simulink model "Flight_simulator_nl"  (R2025b)
settings: Solver=ode4  StartTime=0.0  StopTime=300  FixedStep=0.02  RelTol=1e-3
InitFcn:
  | navion_params;
  | actuator_params;
  | figs0 = findall(0, 'type', 'figure');
  | vis0  = get(0, 'DefaultFigureVisible');
  | set(0, 'DefaultFigureVisible', 'off');
  | evalc('longitudinal_pitch_control; lateral_directional_control;');
  | set(0, 'DefaultFigureVisible', vis0);
  | close(setdiff(findall(0, 'type', 'figure'), figs0));
  | if ~exist('fb_on',   'var'), fb_on   = 1; end
  | if ~exist('gust_on', 'var'), gust_on = 1; end
  | if ~exist('trk_on','var'), trk_on = 1; end
  | nl_setup;
undefined symbols (not defined in the file): act_on, alt_on, F, fb_on, gust_on, Kh, Ki, Kp, Kphi, Kpsi, Kq, Kv, Kvi, Kxi, Ky, Kzeta, Light, MIL, nl_x0, pos_ail, pos_ele, pos_rud, psi_int_lim, sens_on, tau_sens, tau_thr, trk_on, V0
libraries: aerolibactuator x3, slpidlib x2, aerolibwind2 x1
settings Model: Creator=USER  LastModifiedBy=USER

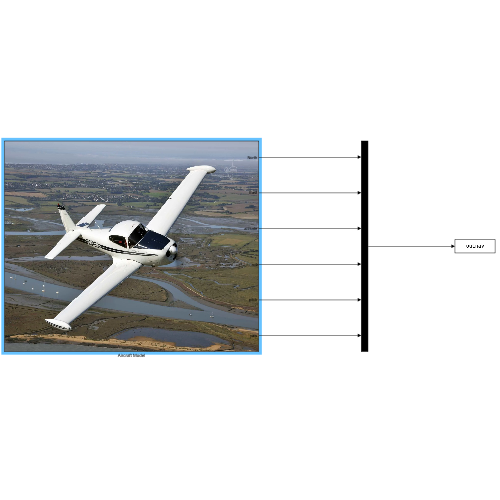
[thumbnail: Simulink's stored preview of the top-level diagram]
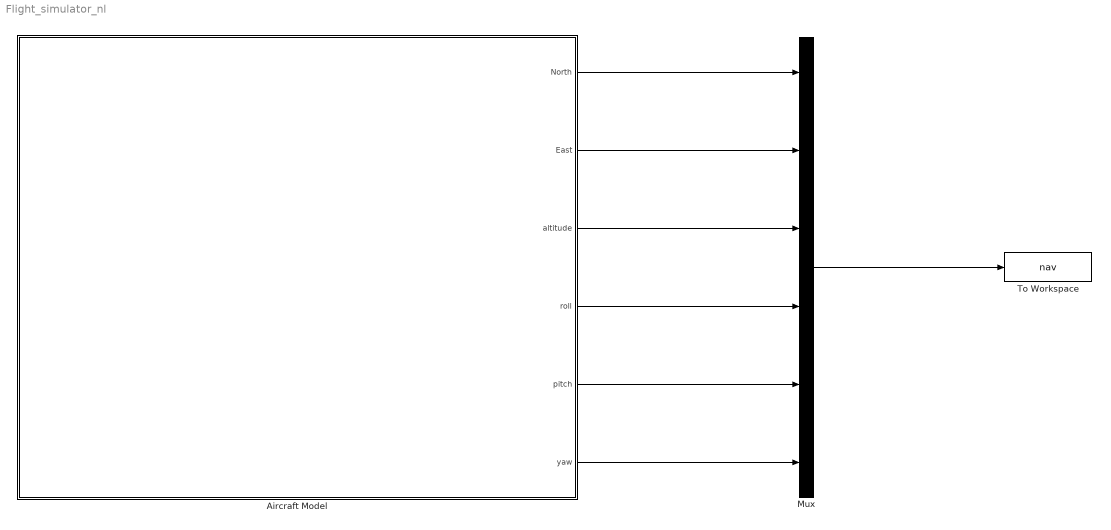
== system Flight_simulator_nl ==
  Aircraft Model : Subsystem
      mask Display: image('img.webp');
  Mux : Mux  Inputs=6
  To Workspace : ToWorkspace  VariableName=nav  SampleTime=-1
  wires:
  Aircraft Model/4(roll) -> Mux/4
  Aircraft Model/5(pitch) -> Mux/5
  Aircraft Model/6(yaw) -> Mux/6
  Aircraft Model/2(East) -> Mux/2
  Aircraft Model/1(North) -> Mux/1
  Aircraft Model/3(altitude) -> Mux/3
  Mux/1 -> To Workspace/1

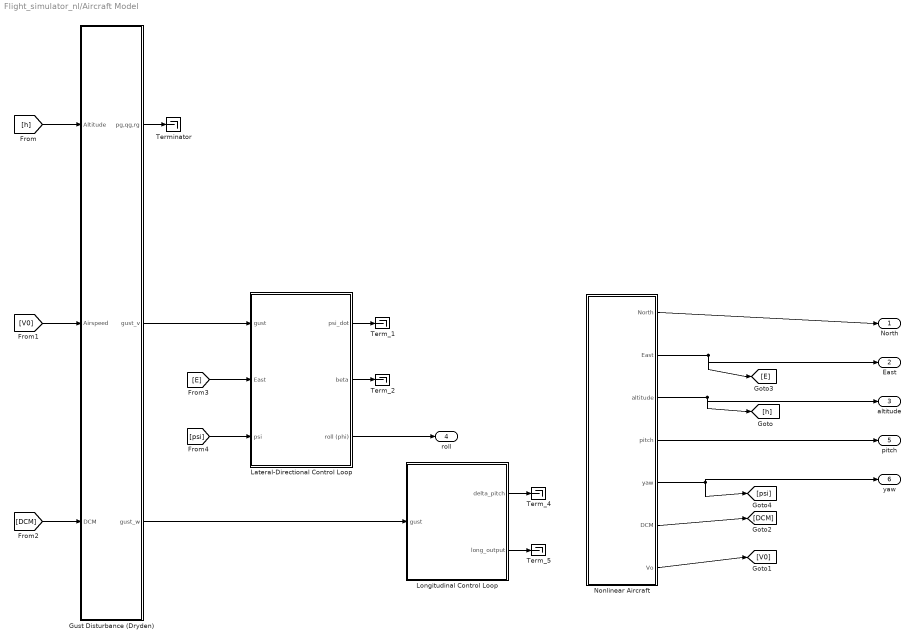
== system Flight_simulator_nl/Aircraft Model ==
  Gust Disturbance (Dryden) : Subsystem
  Lateral-Directional Control Loop : Subsystem
  Longitudinal Control Loop : Subsystem
  Nonlinear Aircraft : Subsystem
  Term_{1..2,4..5} (4 alike) : Terminator
  Terminator : Terminator
  North : Outport
  East : Outport  Port=2
  altitude : Outport  Port=3
  roll : Outport  Port=4
  pitch : Outport  Port=5
  yaw : Outport  Port=6
  wires:
  Gust Disturbance (Dryden)/3(gust_w) -> Longitudinal Control Loop/1(gust)
  [DCM] -> Gust Disturbance (Dryden)/3(DCM)
  [h] -> Gust Disturbance (Dryden)/1(Altitude)
  [V0] -> Gust Disturbance (Dryden)/2(Airspeed)
  Lateral-Directional Control Loop/3(roll (phi)) -> roll/1
  Gust Disturbance (Dryden)/1(pg,qg,rg) -> Terminator/1
  Gust Disturbance (Dryden)/2(gust_v) -> Lateral-Directional Control Loop/1(gust)
  [E] -> Lateral-Directional Control Loop/2(East)
  [psi] -> Lateral-Directional Control Loop/3(psi)
  Lateral-Directional Control Loop/1(psi_dot) -> Term_1/1
  Lateral-Directional Control Loop/2(beta) -> Term_2/1
  Longitudinal Control Loop/1("delta_pitch ") -> Term_4/1
  Longitudinal Control Loop/2(long_output) -> Term_5/1
  Nonlinear Aircraft/1(North) -> North/1
  Nonlinear Aircraft/2(East) -> [E], East/1
  Nonlinear Aircraft/3(altitude) -> [h], altitude/1
  Nonlinear Aircraft/4(pitch) -> pitch/1
  Nonlinear Aircraft/5(yaw) -> [psi], yaw/1
  Nonlinear Aircraft/6(DCM) -> [DCM]
  Nonlinear Aircraft/7(Vo) -> [V0]

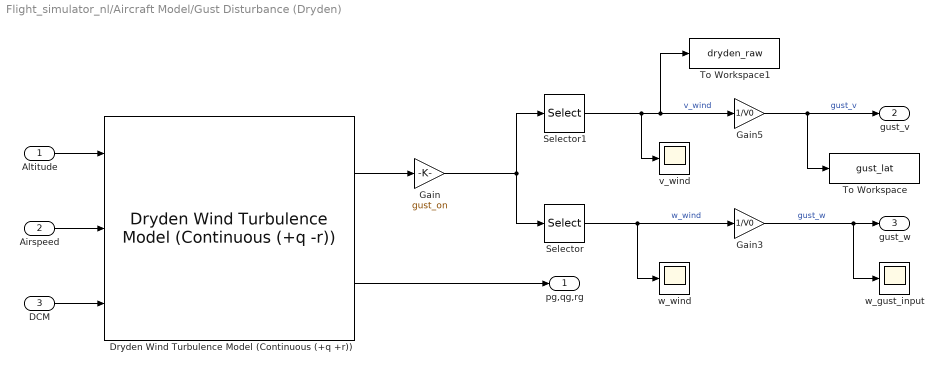
== system Flight_simulator_nl/Aircraft Model/Gust Disturbance (Dryden) ==
  Altitude : Inport
  Airspeed : Inport  Port=2
  DCM : Inport  Port=3
  Dryden Wind Turbulence Model (Continuous (+q +r)) : aerolibwind2/Dryden Wind Turbulence Model  (Continuous (+q -r))  units=Metric (MKS)  spec=MIL-F-8785C  model=Continuous Dryden (+q +r)  W20=15  Wdeg=0  TurbProb=10^-2 - Light  L_high=533.4  Wingspan=10  ts=0.1  Seed=[1010 1011 1012 1013]  T_on=on
      settings: LibrarySourceBlock=|
      | aerolibwind2/Dryden Wind Turbulence Model
      | (Continuous (+q +r))
  Gain : Gain  Gain=gust_on
  Gain3 : Gain  Gain=1/V0
  Gain5 : Gain  Gain=1/V0
  Selector : Selector  InputPortWidth=3  IndexOptions=Index vector (dialog)  Indices=3  OutputSizes=1
  Selector1 : Selector  InputPortWidth=3  IndexOptions=Index vector (dialog)  Indices=2  OutputSizes=1
  To Workspace : ToWorkspace  VariableName=gust_lat  SampleTime=-1
  To Workspace1 : ToWorkspace  VariableName=dryden_raw  SampleTime=-1
  v_wind : Scope
      settings: ActiveDisplayYMinimum=-2.1718299710396272  ActiveDisplayYMaximum=2.2933542366070889  DataLoggingVariableName=ScopeData3
  w_gust_input : Scope
      settings: ActiveDisplayYMinimum=-10.465820831986111  ActiveDisplayYMaximum=10.534179168013885
  w_wind : Scope
      settings: ActiveDisplayYMinimum=-10.465820831986111  ActiveDisplayYMaximum=10.534179168013885  DataLoggingVariableName=ScopeData2
  pg,qg,rg : Outport
  gust_v : Outport  Port=2
  gust_w : Outport  Port=3
  wires:
  Selector1/1 -> v_wind/1, To Workspace1/1, Gain5/1  "v_wind"
  Altitude/1 -> Dryden Wind Turbulence Model (Continuous (+q +r))/1
  Airspeed/1 -> Dryden Wind Turbulence Model (Continuous (+q +r))/2
  Dryden Wind Turbulence Model (Continuous (+q +r))/2 -> pg,qg,rg/1
  DCM/1 -> Dryden Wind Turbulence Model (Continuous (+q +r))/3
  Dryden Wind Turbulence Model (Continuous (+q +r))/1 -> Gain/1
  Selector/1 -> Gain3/1, w_wind/1  "w_wind"
  Gain5/1 -> To Workspace/1, gust_v/1  "gust_v"
  Gain3/1 -> gust_w/1, w_gust_input/1  "gust_w"
  Gain/1 -> Selector/1, Selector1/1

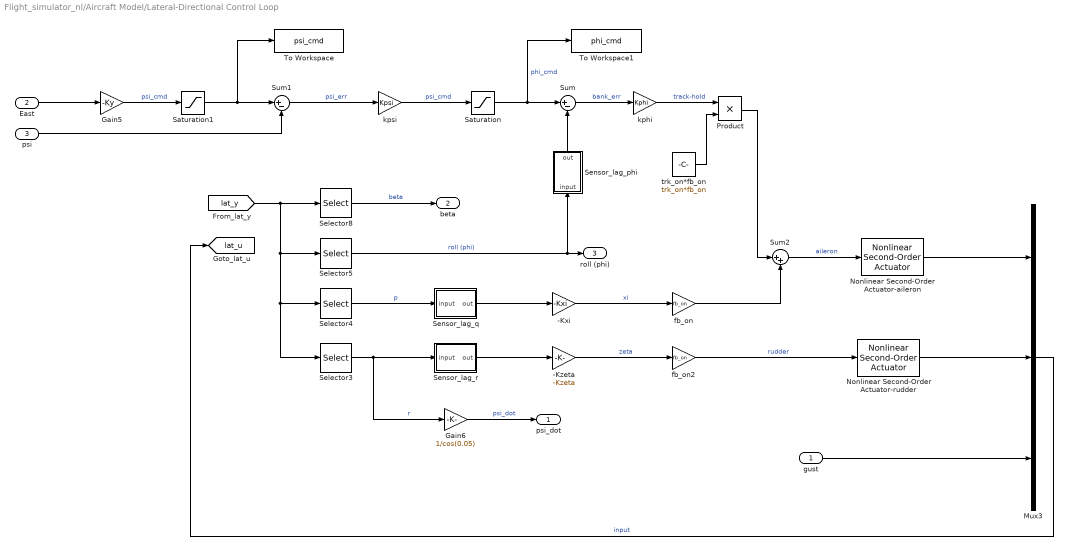
== system Flight_simulator_nl/Aircraft Model/Lateral-Directional Control Loop ==
  gust : Inport
  East : Inport  Port=2
  psi : Inport  Port=3
  -Kxi : Gain  Gain=-Kxi
  -Kzeta : Gain  Gain=-Kzeta
  Gain5 : Gain  Gain=-Ky
  Gain6 : Gain  Gain=1/cos(0.05)
  Mux3 : Mux  Inputs=3
  Nonlinear Second-Order Actuator-aileron : aerolibactuator/Nonlinear Second-Order Actuator  wn_fin=wn_ail  z_fin=zeta_ail  fin_max=pos_ail  fin_min=-pos_ail  fin_maxrate=rate_ail  fin_act_0=0  fin_act_vel=0
  Nonlinear Second-Order Actuator-rudder : aerolibactuator/Nonlinear Second-Order Actuator  wn_fin=wn_rud  z_fin=zeta_rud  fin_max=pos_rud  fin_min=-pos_rud  fin_maxrate=rate_rud  fin_act_0=0  fin_act_vel=0
  Product : Product
  Saturation : Saturate  UpperLimit=0.35  LowerLimit=-0.35
  Saturation1 : Saturate  UpperLimit=psi_int_lim  LowerLimit=-psi_int_lim
  Selector3 : Selector  InputPortWidth=4  IndexOptions=Index vector (dialog)  Indices=1  OutputSizes=1
  Selector4 : Selector  InputPortWidth=4  IndexOptions=Index vector (dialog)  Indices=3  OutputSizes=1
  Selector5 : Selector  InputPortWidth=4  IndexOptions=Index vector (dialog)  Indices=4  OutputSizes=1
  Selector8 : Selector  InputPortWidth=4  IndexOptions=Index vector (dialog)  Indices=2  OutputSizes=1
  Sensor_lag_phi : Subsystem
  Sensor_lag_q : Subsystem
  Sensor_lag_r : Subsystem
  Sum : Sum  Inputs=|+-
  Sum1 : Sum  Inputs=|+-
  Sum2 : Sum  Inputs=|++
  To Workspace : ToWorkspace  VariableName=psi_cmd  SampleTime=-1
  To Workspace1 : ToWorkspace  VariableName=phi_cmd  SampleTime=-1
  fb_on : Gain  Gain=fb_on
  fb_on2 : Gain  Gain=fb_on
  kphi : Gain  Gain=Kphi
  kpsi : Gain  Gain=Kpsi
  trk_on*fb_on : Constant  Value=trk_on*fb_on
  psi_dot : Outport
  beta : Outport  Port=2
  roll (phi) : Outport  Port=3
  tag scope: lat_u=global
  wires:
  Selector4/1 -> Sensor_lag_q/1(input)  "p"
  Gain6/1 -> psi_dot/1  "psi_dot"
  Selector5/1 -> roll (phi)/1, Sensor_lag_phi/1(input)  "roll (phi)"
  Selector8/1 -> beta/1  "beta"
  gust/1 -> Mux3/3
  Selector3/1 -> Gain6/1, Sensor_lag_r/1(input)  "r"
  -Kxi/1 -> fb_on/1  "xi"
  -Kzeta/1 -> fb_on2/1  "zeta"
  fb_on/1 -> Sum2/2
  fb_on2/1 -> Nonlinear Second-Order Actuator-rudder/1  "rudder"
  Gain5/1 -> Saturation1/1  "psi_cmd"
  Sum1/1 -> kpsi/1  "psi_err"
  kpsi/1 -> Saturation/1  "psi_cmd"
  East/1 -> Gain5/1
  Saturation/1 -> To Workspace1/1, Sum/1  "phi_cmd"
  Sum/1 -> kphi/1  "bank_err"
  kphi/1 -> Product/1  "track-hold"
  Sum2/1 -> Nonlinear Second-Order Actuator-aileron/1  "aileron"
  Product/1 -> Sum2/1
  trk_on*fb_on/1 -> Product/2
  psi/1 -> Sum1/2
  Nonlinear Second-Order Actuator-rudder/1 -> Mux3/2
  Sensor_lag_q/1(out) -> -Kxi/1
  Sensor_lag_r/1(out) -> -Kzeta/1
  Sensor_lag_phi/1(out) -> Sum/2
  Nonlinear Second-Order Actuator-aileron/1 -> Mux3/1
  [lat_y] -> Selector8/1, Selector3/1, Selector4/1, Selector5/1
  Mux3/1 -> [lat_u]  "input"
  Saturation1/1 -> To Workspace/1, Sum1/1

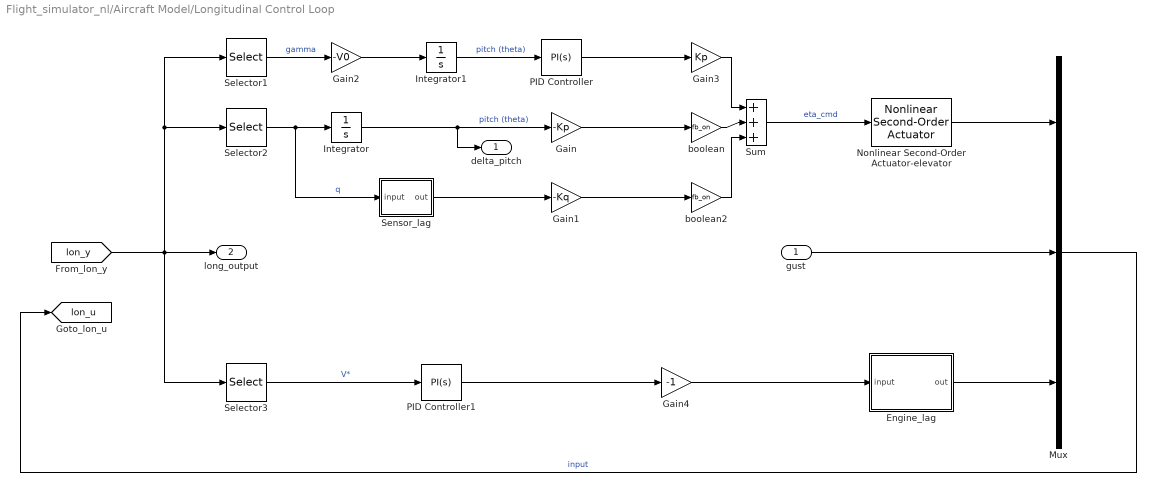
== system Flight_simulator_nl/Aircraft Model/Longitudinal Control Loop ==
  gust : Inport
  Engine_lag : Subsystem  mask{tau=tau_thr, rate_lim=inf, pos_lim=inf}
      mask prompts: tau "Time constant [s]"; rate_lim "Rate limit [rad/s]"; pos_lim "Position limit [rad]"
  Gain : Gain  Gain=-Kp
  Gain1 : Gain  Gain=-Kq
  Gain2 : Gain  Gain=-V0
  Gain3 : Gain  Gain=Kp
  Gain4 : Gain  Gain=-1
  Integrator : Integrator
  Integrator1 : Integrator
  Mux : Mux  Inputs=3
  Nonlinear Second-Order Actuator-elevator : aerolibactuator/Nonlinear Second-Order Actuator  wn_fin=wn_ele  z_fin=zeta_ele  fin_max=pos_ele  fin_min=-pos_ele  fin_maxrate=rate_ele  fin_act_0=0  fin_act_vel=0
  PID Controller : slpidlib/PID Controller  Controller=PI  Form=Parallel  TimeDomain=Continuous-time  UseExternalTs=off  SampleTime=-1  IntegratorMethod=Forward Euler  FilterMethod=Forward Euler  ControllerParametersSource=internal  P=Kh*alt_on  I=Ki*alt_on  UseKiTs=off  D=0  UseExternalDerivativeSource=off  N=100  UseFilter=on  TunerSelectOption=Transfer Function Based (PID Tuner App)  InitialConditionSource=internal  InitialConditionForIntegrator=0  InitialConditionForFilter=0  DifferentiatorICPrevScaledInput=0  ExternalReset=none  TrackingMode=off  Kt=1  LimitOutput=off  SatLimitsSource=internal  UpperSaturationLimit=inf  LowerSaturationLimit=-inf  LinearizeAsGain=on  AntiWindupMode=none  Kb=1  LimitIntegrator=off  UpperIntegratorSaturationLimit=inf  LowerIntegratorSaturationLimit=-inf  POutMin=[]  POutMax=[]  IOutMin=[]  IOutMax=[]  DOutMin=[]  DOutMax=[]  NOutMin=[]  NOutMax=[]  SumOutMin=[]  SumOutMax=[]  SaturationOutMin=[]  SaturationOutMax=[]  PParamMin=[]  PParamMax=[]  IParamMin=[]  IParamMax=[]  DParamMin=[]  DParamMax=[]  NParamMin=[]  NParamMax=[]  KbParamMin=[]  KbParamMax=[]  KtParamMin=[]  KtParamMax=[]  KbOutMin=[]  KbOutMax=[]  KtOutMin=[]  KtOutMax=[]  IntegratorOutMin=[]  IntegratorOutMax=[]  FilterOutMin=[]  FilterOutMax=[]  SumI1OutMin=[]  SumI1OutMax=[]  SumI2OutMin=[]  SumI2OutMax=[]  SumI3OutMin=[]  SumI3OutMax=[]  SumI4OutMin=[]  SumI4OutMax=[]  SumDOutMin=[]  SumDOutMax=[]  DifferentiatorOutMin=[]  DifferentiatorOutMax=[]  FilterDiffOutCoefMin=[]  FilterDiffOutCoefMax=[]  ReciprocalOutMin=[]  ReciprocalOutMax=[]  SumDenOutMin=[]  SumDenOutMax=[]  SumNumOutMin=[]  SumNumOutMax=[]  DivideOutMin=[]  DivideOutMax=[]  UdiffTsProdOutMin=[]  UdiffTsProdOutMax=[]  NTsProdOutMin=[]  NTsProdOutMax=[]  UintegralTsProdOutMin=[]  UintegralTsProdOutMax=[]  UngainTsProdOutMin=[]  UngainTsProdOutMax=[]  ClampingZeroOutDataTypeStr=Inherit: Inherit via back propagation  ClampingZeroOutMin=[]  ClampingZeroOutMax=[]  FilterDenConstantOutDataTypeStr=Inherit: Inherit via back propagation  FilterDenConstantOutMin=[]  FilterDenConstantOutMax=[]  PCopyOutDataTypeStr=Inherit: Inherit via back propagation  PCopyOutMin=[]  PCopyOutMax=[]  NCopyOutDataTypeStr=Inherit: Inherit via back propagation  NCopyOutMin=[]  NCopyOutMax=[]  IntegratorContinuousStateAttributes=''  IntegratorStateMustResolveToSignalObject=off  IntegratorRTWStateStorageClass=Auto  FilterContinuousStateAttributes=''  FilterStateMustResolveToSignalObject=off  FilterRTWStateStorageClass=Auto  ParallelPVariant=InternalParameters  IdealPVariant=Disabled  IVariant=InternalParameters  DVariant=Disabled  IntegratorVariant=Continuous  SatVariant=Disabled  AWVariant=Passthrough  PCopyVariant=Disabled  TRVariant=Disabled  FdbkBlocksVariant=Forward  IdealPFdbkVariant=Disabled  SatFdbkVariant=Disabled  DerivativeFilterVariant=Disabled  NVariant=Disabled  NCopyVariant=Disabled_SignalSpec  FilterICVariant=Disabled  IntegratorICVariant=InternalICs  ExternalResetVariant=Disabled  TRSumVariant=Passthrough  SumFdbkVariant=Disabled  SumVariant=Sum_PI  TsampFilterVariant=InternalTs  TsampNgainVariant=Passthrough  TsampIntegralVariant=Disabled_SignalSpec  ExternalSaturationOutDataTypeStr=Inherit: Same as second input  DerivativeSourceVariant=Disabled  PreIntVariant=InternalPreInt
  PID Controller1 : slpidlib/PID Controller  Controller=PI  Form=Parallel  TimeDomain=Continuous-time  UseExternalTs=off  SampleTime=-1  IntegratorMethod=Forward Euler  FilterMethod=Forward Euler  ControllerParametersSource=internal  P=Kv*alt_on  I=Kvi*alt_on  UseKiTs=off  D=0  UseExternalDerivativeSource=off  N=100  UseFilter=on  TunerSelectOption=Transfer Function Based (PID Tuner App)  InitialConditionSource=internal  InitialConditionForIntegrator=0  InitialConditionForFilter=0  DifferentiatorICPrevScaledInput=0  ExternalReset=none  TrackingMode=off  Kt=1  LimitOutput=off  SatLimitsSource=internal  UpperSaturationLimit=inf  LowerSaturationLimit=-inf  LinearizeAsGain=on  AntiWindupMode=none  Kb=1  LimitIntegrator=off  UpperIntegratorSaturationLimit=inf  LowerIntegratorSaturationLimit=-inf  POutMin=[]  POutMax=[]  IOutMin=[]  IOutMax=[]  DOutMin=[]  DOutMax=[]  NOutMin=[]  NOutMax=[]  SumOutMin=[]  SumOutMax=[]  SaturationOutMin=[]  SaturationOutMax=[]  PParamMin=[]  PParamMax=[]  IParamMin=[]  IParamMax=[]  DParamMin=[]  DParamMax=[]  NParamMin=[]  NParamMax=[]  KbParamMin=[]  KbParamMax=[]  KtParamMin=[]  KtParamMax=[]  KbOutMin=[]  KbOutMax=[]  KtOutMin=[]  KtOutMax=[]  IntegratorOutMin=[]  IntegratorOutMax=[]  FilterOutMin=[]  FilterOutMax=[]  SumI1OutMin=[]  SumI1OutMax=[]  SumI2OutMin=[]  SumI2OutMax=[]  SumI3OutMin=[]  SumI3OutMax=[]  SumI4OutMin=[]  SumI4OutMax=[]  SumDOutMin=[]  SumDOutMax=[]  DifferentiatorOutMin=[]  DifferentiatorOutMax=[]  FilterDiffOutCoefMin=[]  FilterDiffOutCoefMax=[]  ReciprocalOutMin=[]  ReciprocalOutMax=[]  SumDenOutMin=[]  SumDenOutMax=[]  SumNumOutMin=[]  SumNumOutMax=[]  DivideOutMin=[]  DivideOutMax=[]  UdiffTsProdOutMin=[]  UdiffTsProdOutMax=[]  NTsProdOutMin=[]  NTsProdOutMax=[]  UintegralTsProdOutMin=[]  UintegralTsProdOutMax=[]  UngainTsProdOutMin=[]  UngainTsProdOutMax=[]  ClampingZeroOutDataTypeStr=Inherit: Inherit via back propagation  ClampingZeroOutMin=[]  ClampingZeroOutMax=[]  FilterDenConstantOutDataTypeStr=Inherit: Inherit via back propagation  FilterDenConstantOutMin=[]  FilterDenConstantOutMax=[]  PCopyOutDataTypeStr=Inherit: Inherit via back propagation  PCopyOutMin=[]  PCopyOutMax=[]  NCopyOutDataTypeStr=Inherit: Inherit via back propagation  NCopyOutMin=[]  NCopyOutMax=[]  IntegratorContinuousStateAttributes=''  IntegratorStateMustResolveToSignalObject=off  IntegratorRTWStateStorageClass=Auto  FilterContinuousStateAttributes=''  FilterStateMustResolveToSignalObject=off  FilterRTWStateStorageClass=Auto  ParallelPVariant=InternalParameters  IdealPVariant=Disabled  IVariant=InternalParameters  DVariant=Disabled  IntegratorVariant=Continuous  SatVariant=Disabled  AWVariant=Passthrough  PCopyVariant=Disabled  TRVariant=Disabled  FdbkBlocksVariant=Forward  IdealPFdbkVariant=Disabled  SatFdbkVariant=Disabled  DerivativeFilterVariant=Disabled  NVariant=Disabled  NCopyVariant=Disabled_SignalSpec  FilterICVariant=Disabled  IntegratorICVariant=InternalICs  ExternalResetVariant=Disabled  TRSumVariant=Passthrough  SumFdbkVariant=Disabled  SumVariant=Sum_PI  TsampFilterVariant=InternalTs  TsampNgainVariant=Passthrough  TsampIntegralVariant=Disabled_SignalSpec  ExternalSaturationOutDataTypeStr=Inherit: Same as second input  DerivativeSourceVariant=Disabled  PreIntVariant=InternalPreInt
  Selector1 : Selector  InputPortWidth=5  IndexOptions=Index vector (dialog)  Indices=2  OutputSizes=1
  Selector2 : Selector  InputPortWidth=5  IndexOptions=Index vector (dialog)  Indices=4  OutputSizes=1
  Selector3 : Selector  InputPortWidth=5  IndexOptions=Index vector (dialog)  Indices=1  OutputSizes=1
  Sensor_lag : Subsystem
  Sum : Sum  Inputs=|+++
  boolean : Gain  Gain=fb_on
  boolean2 : Gain  Gain=fb_on
  "delta_pitch " : Outport
  long_output : Outport  Port=2
  tag scope: lon_u=global
  wires:
  Selector2/1 -> Sensor_lag/1(input), Integrator/1  "q"
  Integrator/1 -> Gain/1, "delta_pitch "/1  "pitch (theta)"
  Sum/1 -> Nonlinear Second-Order Actuator-elevator/1  "eta_cmd"
  gust/1 -> Mux/2
  Gain1/1 -> boolean2/1
  Gain/1 -> boolean/1
  boolean/1 -> Sum/2
  boolean2/1 -> Sum/3
  Selector1/1 -> Gain2/1  "gamma"
  Gain2/1 -> Integrator1/1
  Integrator1/1 -> PID Controller/1  "pitch (theta)"
  Gain3/1 -> Sum/1
  PID Controller/1 -> Gain3/1
  Selector3/1 -> PID Controller1/1  "V*"
  PID Controller1/1 -> Gain4/1
  Gain4/1 -> Engine_lag/1(input)
  Nonlinear Second-Order Actuator-elevator/1 -> Mux/1
  Engine_lag/1(out) -> Mux/3
  Sensor_lag/1(out) -> Gain1/1
  [lon_y] -> Selector3/1, long_output/1, Selector2/1, Selector1/1
  Mux/1 -> [lon_u]  "input"

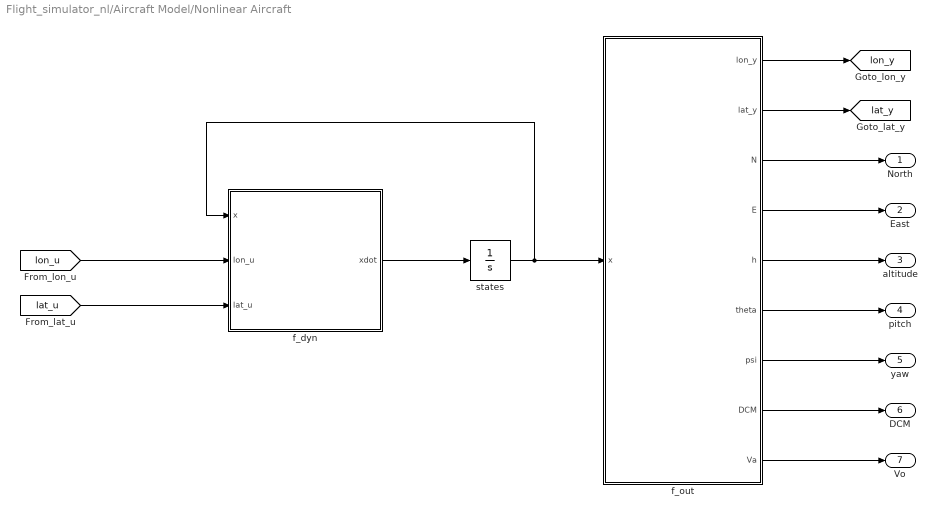
== system Flight_simulator_nl/Aircraft Model/Nonlinear Aircraft ==
  f_dyn : MATLAB Function  TreatAsAtomicUnit=on
  f_out : MATLAB Function  TreatAsAtomicUnit=on
  states : Integrator  InitialCondition=nl_x0
  North : Outport
  East : Outport  Port=2
  altitude : Outport  Port=3
  pitch : Outport  Port=4
  yaw : Outport  Port=5
  DCM : Outport  Port=6
  Vo : Outport  Port=7
  tag scope: lat_y=global, lon_y=global
  wires:
  states/1 -> f_out/1(x), f_dyn/1(x)
  [lon_u] -> f_dyn/2(lon_u)
  [lat_u] -> f_dyn/3(lat_u)
  f_dyn/1(xdot) -> states/1
  f_out/1(lon_y) -> [lon_y]
  f_out/2(lat_y) -> [lat_y]
  f_out/3(N) -> North/1
  f_out/4(E) -> East/1
  f_out/5(h) -> altitude/1
  f_out/6(theta) -> pitch/1
  f_out/7(psi) -> yaw/1
  f_out/8(DCM) -> DCM/1
  f_out/9(Va) -> Vo/1

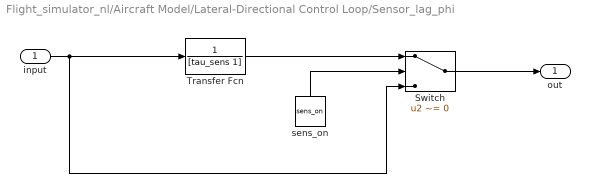
== system Flight_simulator_nl/Aircraft Model/Lateral-Directional Control Loop/Sensor_lag_phi ==
  input : Inport
  Switch : Switch  Criteria=u2 ~= 0  SaturateOnIntegerOverflow=off  InputSameDT=off
  Transfer Fcn : TransferFcn  Denominator=[tau_sens 1]
  sens_on : Constant  Value=sens_on
  out : Outport
  wires:
  Transfer Fcn/1 -> Switch/1
  input/1 -> Transfer Fcn/1, Switch/3
  Switch/1 -> out/1
  sens_on/1 -> Switch/2

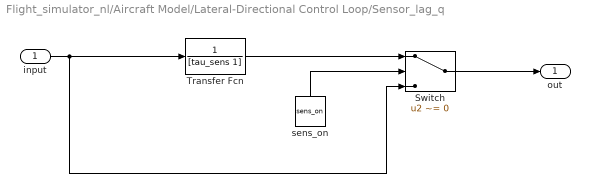
== system Flight_simulator_nl/Aircraft Model/Lateral-Directional Control Loop/Sensor_lag_q ==
  input : Inport
  Switch : Switch  Criteria=u2 ~= 0  SaturateOnIntegerOverflow=off  InputSameDT=off
  Transfer Fcn : TransferFcn  Denominator=[tau_sens 1]
  sens_on : Constant  Value=sens_on
  out : Outport
  wires:
  Transfer Fcn/1 -> Switch/1
  input/1 -> Transfer Fcn/1, Switch/3
  Switch/1 -> out/1
  sens_on/1 -> Switch/2

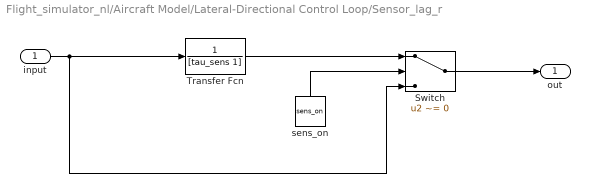
== system Flight_simulator_nl/Aircraft Model/Lateral-Directional Control Loop/Sensor_lag_r ==
  input : Inport
  Switch : Switch  Criteria=u2 ~= 0  SaturateOnIntegerOverflow=off  InputSameDT=off
  Transfer Fcn : TransferFcn  Denominator=[tau_sens 1]
  sens_on : Constant  Value=sens_on
  out : Outport
  wires:
  Transfer Fcn/1 -> Switch/1
  input/1 -> Transfer Fcn/1, Switch/3
  Switch/1 -> out/1
  sens_on/1 -> Switch/2

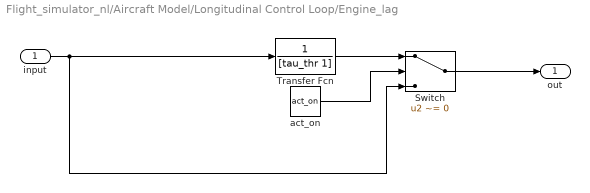
== system Flight_simulator_nl/Aircraft Model/Longitudinal Control Loop/Engine_lag ==
  input : Inport
  Switch : Switch  Criteria=u2 ~= 0  SaturateOnIntegerOverflow=off  InputSameDT=off
  Transfer Fcn : TransferFcn  Denominator=[tau_thr 1]
  act_on : Constant  Value=act_on
  out : Outport
  wires:
  Transfer Fcn/1 -> Switch/1
  input/1 -> Transfer Fcn/1, Switch/3
  Switch/1 -> out/1
  act_on/1 -> Switch/2

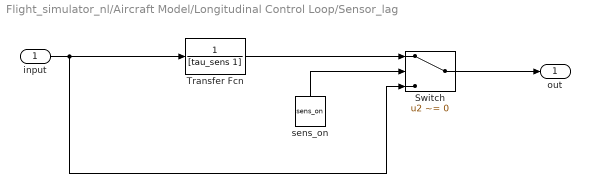
== system Flight_simulator_nl/Aircraft Model/Longitudinal Control Loop/Sensor_lag ==
  input : Inport
  Switch : Switch  Criteria=u2 ~= 0  SaturateOnIntegerOverflow=off  InputSameDT=off
  Transfer Fcn : TransferFcn  Denominator=[tau_sens 1]
  sens_on : Constant  Value=sens_on
  out : Outport
  wires:
  Transfer Fcn/1 -> Switch/1
  input/1 -> Transfer Fcn/1, Switch/3
  Switch/1 -> out/1
  sens_on/1 -> Switch/2

== matlab function Flight_simulator_nl/Aircraft Model/Nonlinear Aircraft/f_out ==
  data: x input size=12; lon_y output size=5; lat_y output size=4; N output size=1; E output size=1; h output size=1; theta output size=1; psi output size=1; DCM output size=[3 3]; Va output size=1
function [lon_y, lat_y, N, E, h, theta, psi, DCM, Va] = f_out(x)
P  = nl_const();
Vg = sqrt(x(1)^2 + x(2)^2 + x(3)^2);
st = sin(x(8)); ct = cos(x(8)); sp = sin(x(7)); cp = cos(x(7)); ss = sin(x(9)); cs = cos(x(9));
Rb2n = [ct*cs, sp*st*cs - cp*ss, cp*st*cs + sp*ss;
        ct*ss, sp*st*ss + cp*cs, cp*st*ss - sp*cs;
        -st,   sp*ct,            cp*ct];
vn    = Rb2n * x(1:3);
gamma = asin(max(-1, min(1, -vn(3)/Vg)));
alpha = atan2(x(3), x(1));
beta  = asin(max(-1, min(1, x(2)/Vg)));
% same layout and meaning as the old state-space outputs (deviations from trim)
lon_y = [Vg - P.V0; gamma; alpha - P.alpha_tr; x(5); x(8) - P.theta_tr];
lat_y = [x(6); beta; x(4); x(7)];
N = x(10); E = x(11); h = x(12); theta = x(8); psi = x(9);
DCM = Rb2n.'; % earth -> body, as the Dryden block expects
Va = Vg;

== matlab function Flight_simulator_nl/Aircraft Model/Nonlinear Aircraft/f_dyn ==
  data: x input size=12; xdot output size=12; lon_u input size=3; lat_u input size=3
function xdot = f_dyn(x, lon_u, lat_u)
% 12-state nonlinear Navion, inputs are deviations from trim
u = [lon_u(1); lat_u(1); lat_u(2); lon_u(3)];   % elevator, aileron, rudder, thrust
g = [lat_u(3); lon_u(2)];                       % beta_g, alpha_g (rad), as the old linear plants
xdot = navion_nl_fcn(x, u, g);
